simulink model "Representacion_en_Espacio_Estados_Simulink"  (R2014a)
settings: Solver=ode45  StartTime=0.0  StopTime=10.0  RelTol=1e-3
values from neighbouring files (symbols this model uses):
  A = [0 1;(-k/m) (-b/m)]    [Representacion_en_Espacio_Estados.m]
  B = 0.5    [Masa_Resorte_Duro_Parametros.m]    (also in Representacion_en_Espacio_Estados.m = [0;(1/m)])
  C = [1 0]    [Representacion_en_Espacio_Estados.m]
settings Model: Creator=Jose  LastModifiedBy=Jose

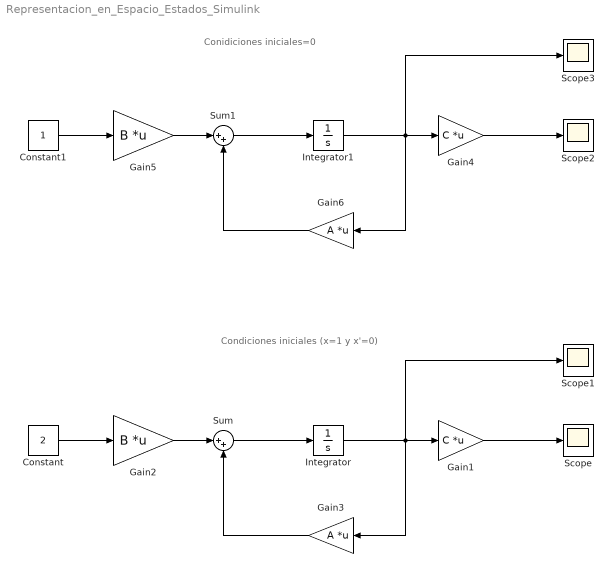
== system Representacion_en_Espacio_Estados_Simulink ==
  note: Conidiciones iniciales=0
  note: Condiciones iniciales (x=1 y x'=0)
  Constant : Constant  Value=2
  Constant1 : Constant
  Gain1 : Gain  Gain=C  Multiplication=Matrix(K*u)
  Gain2 : Gain  Gain=B  Multiplication=Matrix(K*u)
  Gain3 : Gain  Gain=A  Multiplication=Matrix(K*u)
  Gain4 : Gain  Gain=C  Multiplication=Matrix(K*u)
  Gain5 : Gain  Gain=B  Multiplication=Matrix(K*u)
  Gain6 : Gain  Gain=A  Multiplication=Matrix(K*u)
  Integrator : Integrator  InitialCondition=[1;0]
  Integrator1 : Integrator
  Scope{,1..3} (4 alike) : Scope
      Scope2 settings: SaveName=ScopeData2
      Scope3 settings: SaveName=ScopeData3
  Sum : Sum  Inputs=|++
  Sum1 : Sum  Inputs=|++
  wires:
  Gain2/1 -> Sum/1
  Sum/1 -> Integrator/1
  Integrator/1 -> Gain3/1, Scope1/1, Gain1/1
  Gain3/1 -> Sum/2
  Constant/1 -> Gain2/1
  Gain1/1 -> Scope/1
  Gain5/1 -> Sum1/1
  Sum1/1 -> Integrator1/1
  Integrator1/1 -> Gain4/1, Scope3/1, Gain6/1
  Gain6/1 -> Sum1/2
  Constant1/1 -> Gain5/1
  Gain4/1 -> Scope2/1
